simulink subsystem "Triangle_Speed"  (R2022b)
settings: Solver=VariableStepAuto  StartTime=0.0  StopTime=10.0  RelTol=1e-3
libraries: simulink x1
settings Model: Creator=gotta  LastModifiedBy=berti

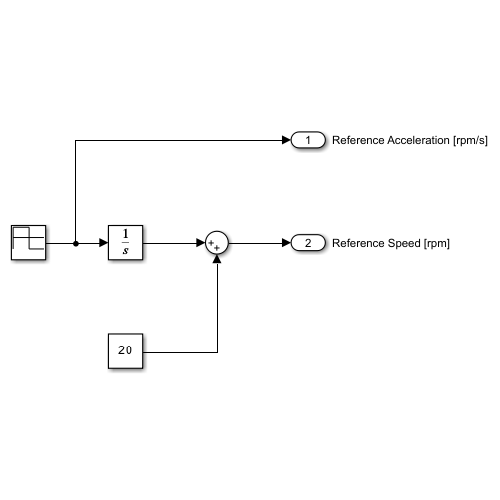
[thumbnail: Simulink's stored preview of the top-level diagram]
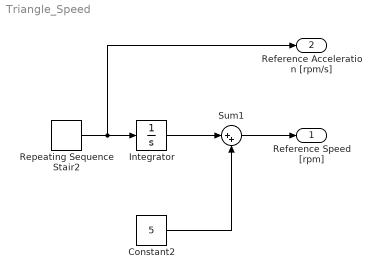
== system Triangle_Speed ==
  Constant2 : Constant  Value=5
  Integrator : Integrator
  Repeating Sequence Stair2 : simulink/Sources/Repeating Sequence Stair  OutValues=4*[10, -10]  tsamp=2.5  OutMin=[]  OutMax=[]  OutDataTypeStr=double  OutputDataTypeScalingMode=double  OutDataType=fixdt(0,8)  ConRadixGroup=Best Precision: Vector-wise  OutScaling=2^-12
  Sum1 : Sum  Inputs=|++
  Reference Speed [rpm] : Outport
  Reference Acceleration [rpm/s] : Outport  Port=2
  wires:
  Constant2/1 -> Sum1/2
  Integrator/1 -> Sum1/1
  Repeating Sequence Stair2/1 -> Reference Acceleration [rpm/s]/1, Integrator/1
  Sum1/1 -> Reference Speed [rpm]/1
